simulink model "V2x_blockset"  (Simulink 7.6)
settings: Solver=ode45  StartTime=0.0  StopTime=10.0  RelTol=1e-3
undefined symbols (not defined in the file or in its folder): intmax, Newton, Raphson
libraries: simulink x53
(part 3 of 3)

== system V2x_blockset/Traffic Controller/Traffic signs and  traffic lights controller/Enabled Subsystem/distance condition/If Action Subsystem1 ==
  headway time : Inport
  d2 : Inport  Port=2
  Action Port : ActionPort  PropagateVarSize=During execution
  Add : Sum
  Gain : Gain  Gain=0
  t2 : Outport
  wires:
  Add/1 -> t2/1
  headway time/1 -> Add/2
  Gain/1 -> Add/1
  d2/1 -> Gain/1

== system V2x_blockset/Traffic Controller/Traffic signs and  traffic lights controller/Enabled Subsystem/major object selection lights/If Action Subsystem ==
  cond : Inport
  messagesID : Inport  Port=2
  traffic lights priorities : Inport  Port=3
  Action Port : ActionPort  PropagateVarSize=During execution
  Reshape1 : Reshape  OutputDimensionality=Column vector (2-D)
  Reshape2 : Reshape  OutputDimensionality=Column vector (2-D)
  Reshape3 : Reshape  OutputDimensionality=Column vector (2-D)
  Selector : Selector  NumberOfDimensions=2  InputPortWidth=3  IndexOptions=Index vector (port),Index vector (dialog)  Indices=[1 3],1  OutputSizes=1,1
  Selector1 : Selector  NumberOfDimensions=2  InputPortWidth=3  IndexOptions=Index vector (port),Index vector (dialog)  Indices=[1 3],1  OutputSizes=1,1
  While Iterator Subsystem : Subsystem  TreatAsAtomicUnit=on
  Message : Outport  InitialOutput=0
  Priority : Outport  Port=2  InitialOutput=0
  wires:
  Selector1/1 -> Priority/1
  Reshape3/1 -> Selector1/1
  traffic lights priorities/1 -> Reshape3/1
  messagesID/1 -> Reshape2/1
  While Iterator Subsystem/1(idx) -> Selector1/2, Selector/2
  Reshape2/1 -> Selector/1
  Reshape1/1 -> While Iterator Subsystem/1(cond)
  Selector/1 -> Message/1
  cond/1 -> Reshape1/1

== system V2x_blockset/Traffic Controller/Traffic signs and  traffic lights controller/Enabled Subsystem/major object selection lights/If Action Subsystem1 ==
  Action Port : ActionPort  PropagateVarSize=During execution
  Constant1 : Constant  Value=0
  Constant2 : Constant  Value=0
  Message : Outport  InitialOutput=0
  Priority : Outport  Port=2  InitialOutput=0
  wires:
  Constant2/1 -> Priority/1
  Constant1/1 -> Message/1

== system V2x_blockset/Traffic Controller/Traffic signs and  traffic lights controller/Enabled Subsystem/major object selection lights/Traffic Lights Warning ==
  trafficLightPriority : Inport
  Data Type Conversion : DataTypeConversion
  Logical Operator : Logic  Operator=OR  AllPortsSameDT=off  OutDataTypeStr=boolean
  if Orange light : simulink/Logic and Bit Operations/Compare To Constant  SystemSampleTime=-1  relop===  const=2  LogicOutDataTypeMode=uint8  ZeroCross=off
  if Red light : simulink/Logic and Bit Operations/Compare To Constant  SystemSampleTime=-1  relop===  const=1  LogicOutDataTypeMode=uint8  ZeroCross=off
  Warning : Outport
  wires:
  trafficLightPriority/1 -> if Orange light/1, if Red light/1
  Data Type Conversion/1 -> Warning/1
  Logical Operator/1 -> Data Type Conversion/1
  if Red light/1 -> Logical Operator/2
  if Orange light/1 -> Logical Operator/1

== system V2x_blockset/Traffic Controller/Traffic signs and  traffic lights controller/Enabled Subsystem/major object selection signs/If Action Subsystem ==
  cond : Inport
  messagesID : Inport  Port=2
  hostVelocity : Inport  Port=3
  Action Port : ActionPort  PropagateVarSize=During execution
  Reshape1 : Reshape  OutputDimensionality=Column vector (2-D)
  Reshape2 : Reshape  OutputDimensionality=Column vector (2-D)
  Selector : Selector  NumberOfDimensions=2  InputPortWidth=3  IndexOptions=Index vector (port),Index vector (dialog)  Indices=[1 3],1  OutputSizes=1,1
  Selector1 : Selector  NumberOfDimensions=2  InputPortWidth=3  IndexOptions=Index vector (port),Index vector (dialog)  Indices=[1 3],1  OutputSizes=1,1
  Traffic signs warning : Subsystem
  While Iterator Subsystem : Subsystem  TreatAsAtomicUnit=on
  Warning : Outport
  Message : Outport  Port=2  InitialOutput=0
  wires:
  Selector1/1 -> Traffic signs warning/1(MessageID)
  Traffic signs warning/1(Warning) -> Warning/1
  hostVelocity/1 -> Traffic signs warning/2(hostVelocity)
  messagesID/1 -> Reshape2/1
  While Iterator Subsystem/1(idx) -> Selector1/2, Selector/2
  Reshape2/1 -> Selector1/1, Selector/1
  Reshape1/1 -> While Iterator Subsystem/1(cond)
  Selector/1 -> Message/1
  cond/1 -> Reshape1/1

== system V2x_blockset/Traffic Controller/Traffic signs and  traffic lights controller/Enabled Subsystem/major object selection signs/If Action Subsystem1 ==
  Action Port : ActionPort  PropagateVarSize=During execution
  Constant1 : Constant  Value=0
  Constant2 : Constant  Value=0
  Warning : Outport  InitialOutput=0
  Message : Outport  Port=2  InitialOutput=0
  wires:
  Constant2/1 -> Warning/1
  Constant1/1 -> Message/1

== system V2x_blockset/Traffic Controller/Traffic signs and  traffic lights controller/Enabled Subsystem/orientation condition/to local reference system ==
  rotZ : Inport
  dX : Inport  Port=2
  dY : Inport  Port=3
  Add : Sum
  Add1 : Sum  Inputs=+-
  Product{,1..3} (4 alike) : Product  RndMeth=Zero
  Trigonometric Function : Trigonometry
  Trigonometric Function1 : Trigonometry  Operator=cos
  dy : Outport
  dx : Outport  Port=2
  wires:
  Add1/1 -> dy/1
  Add/1 -> dx/1
  Product3/1 -> Add1/2
  Product2/1 -> Add1/1
  Product/1 -> Add/2
  Product1/1 -> Add/1
  dY/1 -> Product2/2, Product1/2
  Trigonometric Function/1 -> Product3/1, Product1/1
  dX/1 -> Product3/2, Product/2
  Trigonometric Function1/1 -> Product2/1, Product/1
  rotZ/1 -> Trigonometric Function1/1, Trigonometric Function/1

== system V2x_blockset/Traffic Controller/Traffic signs and  traffic lights controller/Enabled Subsystem/right road side condition/to local reference system ==
  rotZ : Inport
  dX : Inport  Port=2
  dY : Inport  Port=3
  Add1 : Sum  Inputs=+-
  Product2 : Product  RndMeth=Zero
  Product3 : Product  RndMeth=Zero
  Trigonometric Function : Trigonometry
  Trigonometric Function1 : Trigonometry  Operator=cos
  dy : Outport
  wires:
  rotZ/1 -> Trigonometric Function/1, Trigonometric Function1/1
  Trigonometric Function1/1 -> Product2/1
  dX/1 -> Product3/2
  Trigonometric Function/1 -> Product3/1
  dY/1 -> Product2/2
  Product2/1 -> Add1/1
  Product3/1 -> Add1/2
  Add1/1 -> dy/1

== system V2x_blockset/Traffic Controller/Intersection warning controller/Enabled Subsystem/Intersection/Closest crossing selection/GPS to XYZ difference (vectorized) ==
  hostLat : Inport
  hostLong : Inport  Port=2
  hostAlt : Inport  Port=3
  lat : Inport  Port=4
  long : Inport  Port=5
  alt : Inport  Port=6
  Add : Sum  Inputs=+-
  Add1 : Sum  Inputs=+-
  Add2 : Sum  Inputs=+-
  Add3 : Sum  Inputs=+++
  Product{,1..4} (5 alike) : Product  RndMeth=Zero
  d2r : Gain  Gain=pi/180
  d2r1 : Gain  Gain=pi/180
  mean Earth radius (latitudal) : Constant  Value=6335439.8775
  mean Earth radius (longitudal) : Constant  Value=6378137.55
  dist_sq : Outport
  wires:
  lat/1 -> Add/1
  hostLat/1 -> Add/2
  long/1 -> Add1/1
  hostLong/1 -> Add1/2
  alt/1 -> Add2/1
  hostAlt/1 -> Add2/2
  Add/1 -> d2r/1
  Add1/1 -> d2r1/1
  d2r/1 -> Product2/1
  d2r1/1 -> Product1/1
  mean Earth radius (longitudal)/1 -> Product1/2
  mean Earth radius (latitudal)/1 -> Product2/2
  Product2/1 -> Product/1, Product/2
  Product1/1 -> Product3/1, Product3/2
  Add2/1 -> Product4/2, Product4/1
  Product/1 -> Add3/1
  Product3/1 -> Add3/2
  Product4/1 -> Add3/3
  Add3/1 -> dist_sq/1

== system V2x_blockset/Traffic Controller/Intersection warning controller/Enabled Subsystem/Intersection/Closest crossing selection/If Action Subsystem ==
  min : Inport
  dist_sq : Inport  Port=2
  GPS lat1 : Inport  Port=3
  GPS long1 : Inport  Port=4
  GPS alt1 : Inport  Port=5
  Action Port : ActionPort  PropagateVarSize=During execution
  Product7 : Product  RndMeth=Zero
  Product8 : Product  RndMeth=Zero
  Product9 : Product  RndMeth=Zero
  Relational Operator3 : RelationalOperator  Operator===  OutDataTypeStr=boolean
  Sum6 : Sum  Inputs=+
  Sum7 : Sum  Inputs=+
  Sum8 : Sum  Inputs=+
  GPS lat : Outport  InitialOutput=0
  GPS long : Outport  Port=2  InitialOutput=0
  GPS alt : Outport  Port=3  InitialOutput=0
  wires:
  min/1 -> Relational Operator3/1
  dist_sq/1 -> Relational Operator3/2
  Relational Operator3/1 -> Product7/1, Product8/1, Product9/1
  GPS lat1/1 -> Product7/2
  GPS long1/1 -> Product8/2
  GPS alt1/1 -> Product9/2
  Product7/1 -> Sum6/1
  Product8/1 -> Sum7/1
  Product9/1 -> Sum8/1
  Sum6/1 -> GPS lat/1
  Sum7/1 -> GPS long/1
  Sum8/1 -> GPS alt/1

== system V2x_blockset/Traffic Controller/Intersection warning controller/Enabled Subsystem/Intersection/Closest crossing selection/If Action Subsystem1 ==
  Action Port : ActionPort  PropagateVarSize=During execution
  Constant : Constant  Value=0
  Constant1 : Constant  Value=0
  Constant2 : Constant  Value=0
  GPS lat : Outport  InitialOutput=0
  GPS long : Outport  Port=2  InitialOutput=0
  GPS alt : Outport  Port=3  InitialOutput=0
  wires:
  Constant/1 -> GPS lat/1
  Constant1/1 -> GPS long/1
  Constant2/1 -> GPS alt/1

== system V2x_blockset/Traffic Controller/Intersection warning controller/Enabled Subsystem/Intersection/Intersection collision warning controller/For Each Subsystem ==
  actorType : Inport  PortDimensions=1  Partition=on  PartitionDimension=1  PartitionWidth=1
  WM : Inport  Port=2  Partition=off
  Rcross : Inport  Port=3  Partition=off
  target range : Inport  Port=4  Partition=on  PartitionDimension=1  PartitionWidth=1
  target angle : Inport  Port=5  Partition=on  PartitionDimension=1  PartitionWidth=1
  target intention : Inport  Port=6  Partition=on  PartitionDimension=1  PartitionWidth=1
  target heading : Inport  Port=7  Partition=on  PartitionDimension=1  PartitionWidth=1
  targetVelocity : Inport  Port=8  PortDimensions=1  Partition=on  PartitionDimension=1  PartitionWidth=1
  For Each : ForEach  DisableCoverage=on  IndexMode=One-based
  If : If  NumInputs=2  IfExpression=(u1==1 | u1==2 | u1 ==3) & (u2~=0)
  If Action Subsystem : Subsystem  TreatAsAtomicUnit=on
  If Action Subsystem1 : Subsystem  TreatAsAtomicUnit=on
  Merge : Merge
  Merge1 : Merge
  Merge2 : Merge
  warning left lane : Outport  ConcatenationDimension=1
  warning straight lane : Outport  Port=2  ConcatenationDimension=1
  warning right lane : Outport  Port=3  ConcatenationDimension=1
  wires:
  actorType/1 -> If/1
  If/1 -> If Action Subsystem/Action
  If/2 -> If Action Subsystem1/Action
  WM/1 -> If Action Subsystem/1(WM)
  Rcross/1 -> If Action Subsystem/2(Rcross)
  target range/1 -> If Action Subsystem/3(target range)
  target angle/1 -> If Action Subsystem/4(target angle)
  target intention/1 -> If Action Subsystem/5(target intention)
  target heading/1 -> If Action Subsystem/6(target heading)
  If Action Subsystem/1(warning left lane) -> Merge/1
  If Action Subsystem/2(warning straight lane) -> Merge1/1
  If Action Subsystem/3(warning right lane) -> Merge2/1
  If Action Subsystem1/1(warning left lane) -> Merge/2
  If Action Subsystem1/2(warning straight lane) -> Merge1/2
  If Action Subsystem1/3(warning right lane) -> Merge2/2
  Merge/1 -> warning left lane/1
  Merge1/1 -> warning straight lane/1
  Merge2/1 -> warning right lane/1
  targetVelocity/1 -> If/2

== system V2x_blockset/Traffic Controller/Intersection warning controller/Enabled Subsystem/Intersection/Intersection collision warning controller/host intention translation ==
  host intention : Inport
  Bias : Bias  Bias=2
  Multiport Switch : MultiPortSwitch  zeroidx=off
  left_turning : Constant  Value=[0 1 1 1 1 1 0 1 1]
  right_turning : Constant  Value=[0 1 0 0 0 1 0 0 0]
  straight : Constant  Value=[0 1 1 0 0 1 1 1 1]
  WM : Outport
  wires:
  right_turning/1 -> Multiport Switch/4
  straight/1 -> Multiport Switch/3
  left_turning/1 -> Multiport Switch/2
  host intention/1 -> Bias/1
  Bias/1 -> Multiport Switch/1
  Multiport Switch/1 -> WM/1

== system V2x_blockset/Traffic Controller/Traffic signs and  traffic lights controller/Enabled Subsystem/major object selection lights/If Action Subsystem/While Iterator Subsystem ==
  cond : Inport
  Compare To Zero : simulink/Logic and Bit Operations/Compare To Zero  SystemSampleTime=-1  relop===  LogicOutDataTypeMode=uint8  ZeroCross=off
  Selector : Selector  NumberOfDimensions=2  InputPortWidth=3  IndexOptions=Index vector (port),Index vector (dialog)  Indices=[1 3],1  OutputSizes=1,1
  While Iterator : WhileIterator  MaxIters=-1  WhileBlockType=do-while  ShowIterationPort=on  OutputDataType=double
  idx : Outport
  wires:
  Selector/1 -> Compare To Zero/1
  cond/1 -> Selector/1
  While Iterator/1 -> idx/1, Selector/2
  Compare To Zero/1 -> While Iterator/1

== system V2x_blockset/Traffic Controller/Traffic signs and  traffic lights controller/Enabled Subsystem/major object selection signs/If Action Subsystem/Traffic signs warning ==
  MessageID : Inport
  hostVelocity : Inport  Port=2
  Compare To Zero : simulink/Logic and Bit Operations/Compare To Zero  SystemSampleTime=-1  relop=>  LogicOutDataTypeMode=uint8  ZeroCross=off
  Data Type Conversion : DataTypeConversion
  Gain : Gain  Gain=3.6
  Logical Operator : Logic  AllPortsSameDT=off  OutDataTypeStr=boolean
  Relational Operator : RelationalOperator  Operator=<  OutDataTypeStr=boolean
  message to speed limit conversion : Bias  Bias=-1000
  Warning : Outport
  wires:
  Logical Operator/1 -> Data Type Conversion/1
  Compare To Zero/1 -> Logical Operator/1
  Relational Operator/1 -> Logical Operator/2
  Gain/1 -> Relational Operator/2
  hostVelocity/1 -> Gain/1
  message to speed limit conversion/1 -> Compare To Zero/1, Relational Operator/1
  MessageID/1 -> message to speed limit conversion/1
  Data Type Conversion/1 -> Warning/1

== system V2x_blockset/Traffic Controller/Traffic signs and  traffic lights controller/Enabled Subsystem/major object selection signs/If Action Subsystem/While Iterator Subsystem ==
  cond : Inport
  Compare To Zero : simulink/Logic and Bit Operations/Compare To Zero  SystemSampleTime=-1  relop===  LogicOutDataTypeMode=uint8  ZeroCross=off
  Selector : Selector  NumberOfDimensions=2  InputPortWidth=3  IndexOptions=Index vector (port),Index vector (dialog)  Indices=[1 3],1  OutputSizes=1,1
  While Iterator : WhileIterator  MaxIters=-1  WhileBlockType=do-while  ShowIterationPort=on  OutputDataType=double
  idx : Outport
  wires:
  Selector/1 -> Compare To Zero/1
  cond/1 -> Selector/1
  While Iterator/1 -> idx/1, Selector/2
  Compare To Zero/1 -> While Iterator/1

== system V2x_blockset/Traffic Controller/Intersection warning controller/Enabled Subsystem/Intersection/Intersection collision warning controller/For Each Subsystem/If Action Subsystem ==
  WM : Inport
  Rcross : Inport  Port=2
  target range : Inport  Port=3
  target angle : Inport  Port=4
  target intention : Inport  Port=5
  target heading : Inport  Port=6
  Action Port : ActionPort
  Decision Algorithm : Stateflow chart  TreatAsAtomicUnit=on
  warning left lane : Outport  InitialOutput=false(1)
  warning straight lane : Outport  Port=2  InitialOutput=false(1)
  warning right lane : Outport  Port=3  InitialOutput=false(1)
  wires:
  Decision Algorithm/1(wLeft) -> warning left lane/1
  Rcross/1 -> Decision Algorithm/2(Rcross)
  target range/1 -> Decision Algorithm/3(range)
  Decision Algorithm/2(wStraight) -> warning straight lane/1
  target angle/1 -> Decision Algorithm/4(angle)
  target intention/1 -> Decision Algorithm/5(intention)
  Decision Algorithm/3(wRight) -> warning right lane/1
  target heading/1 -> Decision Algorithm/6(heading)
  WM/1 -> Decision Algorithm/1(WM)

== system V2x_blockset/Traffic Controller/Intersection warning controller/Enabled Subsystem/Intersection/Intersection collision warning controller/For Each Subsystem/If Action Subsystem1 ==
  Action Port : ActionPort
  Constant : Constant  Value=false(1)
  Constant1 : Constant  Value=false(1)
  Constant2 : Constant  Value=false(1)
  warning left lane : Outport  InitialOutput=false(1)
  warning straight lane : Outport  Port=2  InitialOutput=false(1)
  warning right lane : Outport  Port=3  InitialOutput=false(1)
  wires:
  Constant/1 -> warning left lane/1
  Constant1/1 -> warning straight lane/1
  Constant2/1 -> warning right lane/1

== matlab function light generator/Lights generator ==
  data: red_time input double; lightID output double; yellow_time input double; green_time input double; time input double; time_delay input double; last_time input double; red output double; yellow output double; green output double; light_time output double; last_time_out output double
function [lightID, red, yellow, green, light_time, last_time_out] = fcn(red_time, yellow_time, green_time, time, time_delay, last_time)
%#eml
time2 = time - last_time + time_delay;
if ((time2) <= green_time)
    green = 1;
    yellow = 0;
    red = 0;
    lightID = 3;
    last_time_out = last_time;
    light_time = green_time - time2;
elseif((time2) <= (green_time+yellow_time))
    green = 0;
    yellow = 1;
    red = 0;
    lightID = 2;
    last_time_out = last_time;
    light_time = yellow_time - (time2 - green_time);
elseif((time2) <= (green_time+yellow_time + red_time - yellow_time))
    green = 0;
    yellow = 0;
    red = 1;
    lightID = 1;
    last_time_out = last_time;
    light_time = red_time - (time2 - green_time - yellow_time);
elseif((time2) <= (green_time+yellow_time + red_time))
    green = 0;
    yellow = 1;
    red = 1;
    lightID = 1;
    last_time_out = last_time;
    light_time = red_time - (time2 - green_time - yellow_time);
else
    green = 1;
    yellow = 0;
    red = 0;
    lightID = 3;
    last_time_out = time + time_delay;
    light_time = green_time - (time2 - green_time - yellow_time - red_time);
end

== stateflow chart Traffic Controller/Intersection warning controller/Enabled Subsystem/Intersection/Intersection collision warning controller/For Each Subsystem/If Action Subsystem/Decision Algorithm ==
  state controller
    state Lane3
      state Straight
        en: wRight=WM[8];
      state RightTurn
        en: wRight=WM[7];
      state LeftTurn
        en: wRight=WM[9];
      (junction 36) -> controller.Lane3.LeftTurn [order 2] : [intention<0]
      (junction 36) -> controller.Lane3.Straight [order 3] : [intention==0]
      (default) -> (junction 36) [order 1]
      (default) -> controller.Lane3.Straight [order 2]
      (junction 36) -> controller.Lane3.RightTurn [order 1] : [intention>0]
    state Lane2
      state RightTurn
        en: wStraight=WM[4];
      state LeftTurn
        en: wStraight=WM[6];
      state Straight
        en: wStraight=WM[5];
      (junction 35) -> controller.Lane2.Straight [order 2] : [intention==0]
      (default) -> controller.Lane2.Straight [order 2]
      (junction 35) -> controller.Lane2.RightTurn [order 3] : [intention>0]
      (junction 35) -> controller.Lane2.LeftTurn [order 1] : [intention<0]
      (default) -> (junction 35) [order 1]
    state Lane1
      state Straight
        en: wLeft=WM[2];
      state LeftTurn
        en: wLeft=WM[3];
      state RightTurn
        en: wLeft=WM[1];
      (junction 34) -> controller.Lane1.RightTurn [order 3] : [intention>0]
      (junction 34) -> controller.Lane1.LeftTurn [order 1] : [intention<0]
      (junction 34) -> controller.Lane1.Straight [order 2] : [intention==0]
      (default) -> controller.Lane1.Straight [order 2]
      (default) -> (junction 34) [order 1]
    state Enter
    controller.Lane1.LeftTurn -> Enter
    controller.Lane3.RightTurn -> Enter
    (default) -> Enter : {wLeft=0;
        | wStraight=0;
        | wRight=0;}
    controller.Lane3.Straight -> Enter
    controller.Lane3.LeftTurn -> Enter
    Enter -> Enter [order 4] : {wLeft=0;
        | wStraight=0;
        | wRight=0;}
    controller.Lane1.RightTurn -> Enter
    Enter -> Lane3 [order 2] : [angle>-90 && angle<-45 && range<Rcross...
        | && (heading>45 && heading<135)]
    controller.Lane1.Straight -> Enter
    controller.Lane2.RightTurn -> Enter
    controller.Lane2.LeftTurn -> Enter
    Enter -> Lane2 [order 1] : [angle>0 && angle<45 && range<Rcross...
        | && heading>135 && heading<225]
    Enter -> Lane1 [order 3] : [angle>90 && angle<135 && range<Rcross...
        | && heading>225 && heading<315]
    controller.Lane2.Straight -> Enter
  data: WM input double size=9; Rcross input double; range input double; angle input double; intention input double; heading input double; wLeft output boolean size=1 =false(1); wStraight output boolean size=1 =false(1); wRight output boolean size=1 =false(1)

== matlab function Traffic Controller/Intersection warning controller/Enabled Subsystem/sort using ID/Embedded MATLAB Function ==
  data: y output double; ids input double
function y = fcn(ids)
% Sorts ID vector

[~,y] = sort(ids,'descend');

end

== matlab function EEB/Angle mod ==
  data: u input double; y output double
function y = fcn(u)
%#eml

y = mod(u, 360);

== matlab function Rx_Noise/For Iterator Subsystem/Embedded MATLAB Function ==
  data: CAM input double; CAM_o output double size=[5, 16]; i input double; NoMM input double; tmp_in input double; tmp_out output double
function [CAM_o, tmp_out] = con(CAM, i, NoMM, tmp_in)
%#eml
CAM_o = CAM;
tmp_out = tmp_in;
if (CAM(i, 3) ~= 0)
    if (mod(tmp_in(i), NoMM+1) ~= 0)
        CAM_o(i, :) = zeros(1, 16);
    end
    tmp_out(i) = tmp_in(i)+1;
end

== stateflow chart EEB/EEBL ==
  state EEBL [parallel]
    settings: executionOrder=1
    state vForward
      (junction 119) -> (junction 115) : {bend = 1;}
      (junction 111) -> (junction 116) [order 2] : {bend = 0;}
      (junction 113) -> (junction 133) [order 1] : [(abs(CAM_Heading[i]-selfHeading)<45 || abs(CAM_Heading[i]-selfHeading)>315) || bend == 1 ]
      (default) -> (junction 111)
      (junction 110) -> (junction 116)
      (junction 115) -> (junction 110)
      (junction 129) -> (junction 125) : {vForward = 0;}
      (junction 127) -> (junction 126) : {vForward = 1;}
      (junction 128) -> (junction 127) [order 1] : [((abs(vAngle-selfHeading)<45 || abs(vAngle-selfHeading)>315) && (abs(vDistance*sin(vAngle*d2r))<5.25)) || bend == 1]
      (junction 128) -> (junction 129) [order 2]
      (junction 130) -> (junction 128)
      (junction 132) -> (junction 129)
      (junction 131) -> (junction 130) [order 1] : [vDistance < 100 && (abs(selfGPSAltitude - CAM_GPSAltitude[i]) < 10)]
      (junction 131) -> (junction 132) [order 2]
      (junction 133) -> (junction 131)
      (junction 113) -> (junction 132) [order 2]
      (junction 118) -> (junction 119) [order 1] : [((abs(L/selfVelocity*selfYawRate + selfHeading - CAM_Heading[i]) < 45) || (abs(L/selfVelocity*selfYawRate + selfHeading - CAM_Heading[i]) > 315)) ]
      (junction 116) -> (junction 113)
      (junction 118) -> (junction 110) [order 2] : {bend = 2;}
      (junction 111) -> (junction 112) [order 1] : [((CAM_YawRate[i] > 2 || CAM_YawRate[i] <-2)  && (selfYawRate > 2 || selfYawRate < -2))]
      (junction 112) -> (junction 118) : {R1 = CAM_Velocity[i]/(CAM_YawRate[i]*d2r);
          | R2 = selfVelocity/(selfYawRate*d2r);
          | alfa = CAM_Heading[i]-selfHeading;
          | L = 2*d2r*180*R2*(alfa/360);}
    state dvBreaking
      (junction 122) -> (junction 120)
      (junction 123) -> (junction 121) : {vBreaking = 1;}
      (junction 121) -> (junction 122)
      (junction 124) -> (junction 122) [order 2]
      (junction 124) -> (junction 123) [order 1] : [ (vForward == 1 && CAM_Acceleration[i] < -brakingWarning)]
      (default) -> (junction 124) : /* Velocity */
    state VehicleAngleandDistance
      state vDistance [parallel]
        settings: executionOrder=2
        (junction 140) -> (junction 139) : {c=2*atan2(sqrt(a), sqrt(1-a));}
        (junction 139) -> (junction 114) : {vDistance = 6371000*c;}
        (default) -> (junction 140) : {a = (sin((CAM_GPSLatitude[i]*d2r-selfGPSLatitude*d2r)/2 ))^2+ cos(selfGPSLatitude*d2r)*cos(CAM_GPSLatitude[i]*d2r)*(sin((CAM_GPSLongitude[i]*d2r-selfGPSLongitude*d2r)/2))^2;}
      state vAngle [parallel]
        settings: executionOrder=1
        (default) -> (junction 117) : {vAngle = (atan2(CAM_GPSLatitude[i]-selfGPSLatitude, CAM_GPSLongitude[i] - selfGPSLongitude))/d2r;}
    state Breaking
      (default) -> (junction 135)
      (junction 135) -> (junction 134) : {Breaking = vBreaking;}
    vForward -> dvBreaking
    VehicleAngleandDistance -> vForward
    (junction 136) -> (junction 138) : {i++;}
    Breaking -> (junction 137)
    (junction 137) -> (junction 138) : {i = 0;
        | vBreaking = 0;
        | vForward = 0;}
    dvBreaking -> (junction 136)
    (junction 138) -> Breaking [order 2]
    (junction 138) -> VehicleAngleandDistance [order 1] : [i < CAM_Size && vBreaking != 1 ]
    (default) -> (junction 138) : {i =0;
        | vForward = 0;}
  note: EEB works with continous signal and checks deceleration of vehicles ahead
  data: a local double; alfa local double; bend local double; c local double; i local double; L local double; vAngle local double; vDistance local double; vForward local double; R1 local double; R2 local double; selfGPSLatitude input double; selfGPSLongitude input double; selfGPSAltitude input double; selfHeading input double; selfVelocity input double; selfYawRate input double; CAM_Velocity input double; CAM_Acceleration input double; CAM_YawRate input double; CAM_GPSLatitude input double; CAM_GPSLongitude input double; CAM_GPSAltitude input double; CAM_Heading input double; CAM_Size input double; d2r constant double =pi()/180; Breaking output double; vBreaking local double; brakingWarning constant double =0.4*9.81

== matlab function Rx_Noise/Embedded MATLAB Function ==
  data: CAM_warning input double; CAM output double; CAM_messageID input double; CAM_vehicleID input double; CAM_vehicleType input double; CAM_publicVehicleType input double; CAM_lightBarInUse input double; CAM_sireneInUse input double; CAM_velocity input double; CAM_acceleration input double; CAM_yawRate input double; CAM_turnAdvice input double; CAM_trafficLightPriority input double; CAM_GPSlat input double; CAM_GPSlong input double; CAM_GPSalt input double; CAM_rotZ input double
function CAM = fcn(CAM_warning, CAM_messageID, CAM_vehicleID, CAM_vehicleType, CAM_publicVehicleType, CAM_lightBarInUse, CAM_sireneInUse, CAM_velocity, CAM_acceleration, CAM_yawRate, CAM_turnAdvice, CAM_trafficLightPriority, CAM_GPSlat, CAM_GPSlong, CAM_GPSalt, CAM_rotZ)
%#eml

CAM = [CAM_warning, CAM_messageID, CAM_vehicleID, CAM_vehicleType, CAM_publicVehicleType, CAM_lightBarInUse, CAM_sireneInUse, CAM_velocity, CAM_acceleration, CAM_yawRate, CAM_turnAdvice, CAM_trafficLightPriority, CAM_GPSlat, CAM_GPSlong, CAM_GPSalt, CAM_rotZ];

== matlab function Rx_Noise/Embedded MATLAB Function1 ==
  data: CAM_warning output double; CAM input double; CAM_messageID output double; CAM_vehicleID output double; CAM_vehicleType output double; CAM_publicVehicleType output double; CAM_lightBarInUse output double; CAM_sireneInUse output double; CAM_velocity output double; CAM_acceleration output double; CAM_yawRate output double; CAM_turnAdvice output double; CAM_trafficLightPriority output double; CAM_GPSlat output double; CAM_GPSlong output double; CAM_GPSalt output double; CAM_rotZ output double
function [CAM_warning, CAM_messageID, CAM_vehicleID, CAM_vehicleType, CAM_publicVehicleType, CAM_lightBarInUse, CAM_sireneInUse, CAM_velocity, CAM_acceleration, CAM_yawRate, CAM_turnAdvice, CAM_trafficLightPriority, CAM_GPSlat, CAM_GPSlong, CAM_GPSalt, CAM_rotZ] = fcn(CAM)
%#eml

CAM_warning = CAM(:, 1);
CAM_messageID = CAM(:, 2); 
CAM_vehicleID = CAM(:, 3);
CAM_vehicleType = CAM(:, 4);
CAM_publicVehicleType = CAM(:, 5);
CAM_lightBarInUse = CAM(:, 6);
CAM_sireneInUse = CAM(:, 7);
CAM_velocity = CAM(:, 8);
CAM_acceleration = CAM(:, 9);
CAM_yawRate = CAM(:, 10);
CAM_turnAdvice = CAM(:, 11);
CAM_trafficLightPriority = CAM(:, 12);
CAM_GPSlat = CAM(:, 13);
CAM_GPSlong = CAM(:, 14);
CAM_GPSalt = CAM(:, 15);
CAM_rotZ = CAM(:, 16);

== matlab function GLOSA/Embedded MATLAB Function ==
  data: u input double; y output double
function y = fcn(u)
%#eml

y = mod(u, 360);

== stateflow chart GLOSA/GLOSA ==
  state GLOSA [parallel]
    settings: executionOrder=1
    state dvVelocity
      (default) -> (junction 337) : /* Velocity */
      (junction 337) -> (junction 339) [order 1] : [ (vForward == 1)]
      (junction 339) -> (junction 349) : {dvVelocity = CAM_Velocity[i];}
          | /* If car is at the front desired velocity if cars are set to its value */
      (junction 337) -> (junction 283) [order 2] : {dvVelocity = desiredVelocity;}
      (junction 349) -> (junction 283)
      (junction 283) -> (junction 350)
    state AngleandDistance
      state vDistance [parallel]
        settings: executionOrder=2
        (junction 331) -> (junction 330) : {Distance = 6371000*c;}
            | /*Calculate distance to the object */
        (default) -> (junction 332) : {a = (sin((CAM_GPSLatitude[i]*d2r-selfGPSLatitude*d2r)/2 ))^2+ cos(selfGPSLatitude*d2r)*cos(CAM_GPSLatitude[i]*d2r)*(sin((CAM_GPSLongitude[i]*d2r-selfGPSLongitude*d2r)/2))^2;}
        (junction 332) -> (junction 331) : {c=2*atan2(sqrt(a), sqrt(1-a));}
      state vAngle [parallel]
        settings: executionOrder=1
        (default) -> (junction 333) : {Angle = (atan2(CAM_GPSLatitude[i]-selfGPSLatitude, CAM_GPSLongitude[i] - selfGPSLongitude))/d2r;}
            | /* Calculate angle to the object */
    state diVelocity
      (default) -> (junction 304) : /* Velocity */
      (junction 285) -> (junction 338)
      (junction 304) -> (junction 303) [order 1] : [ (iForward == 1)]
      (junction 304) -> (junction 285) [order 2] : {diVelocity = desiredVelocity;}
      (junction 303) -> (junction 336) : {diVelocity = (CAM_message[i] - 1000) /3.6;}
          | /* If sign is foreward, set desired infrastructure velocity to its limit */
      (junction 336) -> (junction 285)
    state vForward
      (junction 289) -> (junction 295) [order 1] : [((CAM_YawRate[i] > 2 || CAM_YawRate[i] <-2)  && (selfYawRate > 2 || selfYawRate < -2))]
      (junction 295) -> (junction 319) : {R1 = CAM_Velocity[i]/(CAM_YawRate[i]*d2r);
          | R2 = selfVelocity/(selfYawRate*d2r);
          | alfa = CAM_Heading[i]-selfHeading;
          | L = 2*d2r*180*R2*(alfa/360);}
      (junction 356) -> (junction 341)
      (junction 340) -> (junction 356) : {bend = 1;}
          | /* Cars are on the same bent if both have non-zero yaw rate and estimated agle at detected distance of the host car is similar to the angle of detected vehicle */
      (junction 319) -> (junction 341) [order 2] : {bend = 2;}
      (junction 279) -> (junction 282)
      (junction 293) -> (junction 280) [order 2]
      (junction 341) -> (junction 294)
      (junction 294) -> (junction 293)
      (junction 282) -> (junction 280) [order 2]
      (default) -> (junction 289)
      (junction 286) -> (junction 287) [order 1] : [abs((Angle-selfHeading)%%360)<45 || abs((Angle-selfHeading)%%360)>315 || bend == 1]
      (junction 335) -> (junction 327) : {vForward = 0;}
      (junction 287) -> (junction 288) : {vForward = 1;}
          | /* Car is at the front if it will be reached in 2s and angles of cars are similar or they are on the bend */
      (junction 293) -> (junction 279) [order 1] : [(abs(CAM_Heading[i]-selfHeading)<45 || abs(CAM_Heading[i]-selfHeading)>315) || bend == 1 ]
      (junction 286) -> (junction 335) [order 2]
      (junction 282) -> (junction 284) [order 1] : [Distance < 100 && (selfVelocity - CAM_Velocity[i]) > 0 &&((Distance / (selfVelocity - CAM_Velocity[i])) < 2) && (abs(selfGPSAltitude - CAM_GPSAltitude[i]) < 10)]
      (junction 289) -> (junction 294) [order 2] : {bend = 0;}
      (junction 284) -> (junction 286)
      (junction 280) -> (junction 335)
      (junction 319) -> (junction 340) [order 1] : [((abs(L/selfVelocity*selfYawRate + selfHeading - CAM_Heading[i]) < 45) || (abs(L/selfVelocity*selfYawRate + selfHeading - CAM_Heading[i]) > 315)) ]
    state Velocity
      (junction 309) -> (junction 307) [order 2]
      (junction 309) -> (junction 308) [order 1] : [(dvVelocity<diVelocity) && (dvVelocity < desiredVelocity) && (vForward == 1)]
      (junction 311) -> (junction 309)
      (junction 310) -> (junction 311)
      (junction 325) -> (junction 310) : {Velocity = diVelocity;}
          | /* When Velocity from the sign is smaller then actual velocity of the car, Desired host velocity is set to the sign limit */
      (junction 326) -> (junction 311) [order 2] : {Velocity = desiredVelocity;}
      (junction 326) -> (junction 325) [order 1] : [(diVelocity<desiredVelocity)]
      (default) -> (junction 326) : /* Velocity */
      (junction 308) -> (junction 306) : {Velocity = dvVelocity;}
          | /* When detected car hes smaller velocity then host car and sign limits, desired velocity of host car is set to velocity of detected car */
      (junction 307) -> (junction 305) : {Velocity = min(dvVelocity, diVelocity, dlVelocity, desiredVelocity);}
      (junction 306) -> (junction 307)
    state lForward
      note: IF condition1 THEN action1
          | ELSE action2
          | ENDIF
      (junction 346) -> (junction 291) : {lForward = 0;}
      (junction 362) -> (junction 292) : {lForward = 1;}
          | /* Light recognized as foreward one, when it is less then 500m away and Angle to it less then 45 deg.*/
      (junction 344) -> (junction 362) [order 1] : [abs((Angle-selfHeading) %% 360)<45 || abs((Angle-selfHeading)%% 360)>315]
      (junction 344) -> (junction 346) [order 2]
      (junction 359) -> (junction 342) [order 2]
      (junction 343) -> (junction 342) [order 2]
      (junction 348) -> (junction 344)
      (junction 358) -> (junction 343)
      (junction 343) -> (junction 348) [order 1] : [Distance < 500 && (abs(selfGPSAltitude - CAM_GPSAltitude[i]) < 10)]
      (junction 342) -> (junction 346)
      (junction 359) -> (junction 358) [order 1] : [abs(CAM_Heading[i]-selfHeading)<45 || abs(CAM_Heading[i]-selfHeading)>315]
      (default) -> (junction 359)
    state iForward
      note: IF condition1 THEN action1
          | ELSE action2
          | ENDIF
      (junction 281) -> (junction 328) [order 1] : [Distance < 20 && (abs(selfGPSAltitude - CAM_GPSAltitude[i]) < 10)]
      (junction 290) -> (junction 316) [order 1] : [abs((Angle-selfHeading)%%360)<45 || abs((Angle-selfHeading)%%360)>315]
      (junction 281) -> (junction 315) [order 2]
      (junction 316) -> (junction 317) : {iForward = 1;}
          | /* Sign recognized as foreward one, when it is less then 20m away and Angle to it less then 45 deg.*/
      (junction 315) -> (junction 329)
      (junction 328) -> (junction 290)
      (junction 329) -> (junction 318) : {iForward = 0;}
      (junction 290) -> (junction 329) [order 2]
      (junction 334) -> (junction 324) [order 1] : [abs(CAM_Heading[i]-selfHeading)<45 || abs(CAM_Heading[i]-selfHeading)>315]
      (default) -> (junction 334)
      (junction 324) -> (junction 281)
      (junction 334) -> (junction 315) [order 2]
    state dlVelocity
      (junction 322) -> (junction 320) : {dlVelocity = max((Distance-7)/(CAM_warning[i]+20), 0);}
          | /*dlVelocity = Distance/CAM_warning[i];}*/
      (junction 353) -> (junction 323) [order 2]
      (junction 357) -> (junction 360)
      (junction 361) -> (junction 357)
      (junction 351) -> (junction 357) [order 2] : {dlVelocity=desiredVelocity;}
      (junction 347) -> (junction 345)
      (junction 355) -> (junction 353) [order 2]
      (junction 320) -> (junction 361)
      (junction 323) -> (junction 322) [order 2]
      (junction 323) -> (junction 321) [order 1] : [TTL<CAM_warning[i]]
      (junction 355) -> (junction 354) [order 1] : [CAM_trafficLightPriority[i] == 3]
      (junction 321) -> (junction 345) : {dlVelocity= desiredVelocity;}
      (junction 297) -> (junction 347)
      (junction 345) -> (junction 320)
      (junction 354) -> (junction 297) : {dlVelocity=desiredVelocity;}
      (junction 296) -> (junction 347) : {dlVelocity = max((Distance-2)/(CAM_warning[i]+0.5), 0);}
      (junction 353) -> (junction 296) [order 1] : [CAM_trafficLightPriority[i] == 1]
      (default) -> (junction 351) : /* Velocity */
      (junction 351) -> (junction 352) [order 1] : [ lForward == 1]
      (junction 352) -> (junction 355) : {TTL = Distance/selfVelocity;
          | Light = CAM_trafficLightPriority[i];
          | Time = CAM_warning[i];}
    lForward -> dlVelocity
    (junction 299) -> AngleandDistance
    (default) -> (junction 298) : {i =0;
        | vForward = 0;
        | iForward = 0;}
    (junction 298) -> (junction 299) [order 1] : [(vForward ==0 || iForward == 0) && i < CAM_Size]
        |  /*till sign and vehicle aren't detected*/
    (junction 300) -> iForward [order 2] : [iForward == 0 && (CAM_vehicleType[i] == 14 || CAM_vehicleType[i] == 15) && CAM_message[i] > 1000]
        | /* If no traffic sign are detected and Velocity of the sign isn't 0 */
    (junction 302) -> (junction 298) : {i = 0;
        | vForward = 0;
        | iForward = 0;
        | lForward = 0;}
    (junction 312) -> (junction 298) : {i++;}
    (junction 300) -> (junction 301) [order 3]
    (junction 298) -> Velocity [order 2]
    (junction 301) -> vForward [order 1] : [vForward == 0 && CAM_vehicleType[i] != 0]
        | /* If there was no nearer car at the front and Vehicle Type ID isn't 0 */
    (junction 301) -> (junction 312) [order 2]
    iForward -> diVelocity
    Velocity -> (junction 302)
    vForward -> dvVelocity
    dvVelocity -> (junction 314)
    diVelocity -> (junction 314)
    (junction 313) -> (junction 312)
    (junction 314) -> (junction 313)
    AngleandDistance -> (junction 300)
    (junction 300) -> lForward [order 1] : [lForward == 0 && CAM_trafficLightPriority[i] !=0]
    dlVelocity -> (junction 314)
  note: GLOSA Algorithms Based on CAM signal changed to continous
  data: R1 local double; R2 local double; a local double; alfa local double; bend local double; c local double; diVelocity local double =100; dvVelocity local double =100; i local double; iForward local double; L local double; vForward local double; dlVelocity local double =100; selfHeading input double; selfGPSLongitude input double; selfGPSLatitude input double; selfGPSAltitude input double; selfYawRate input double; selfVelocity input double; CAM_warning input double; CAM_message input double; CAM_vehicleType input double; Velocity output double; CAM_Velocity input double; CAM_YawRate input double; CAM_trafficLightPriority input double; CAM_GPSLatitude input double; CAM_GPSLongitude input double; CAM_GPSAltitude input double; CAM_Heading input double; CAM_Size input double; d2r constant double =pi()/180; desiredVelocity input double; TTL local double; lForward output double; Angle local double; Distance local double; Time output double; Light output double

== matlab function GLOSA/vehicle CAM generator/For Iterator Subsystem/Continuous signal ==
  data: CAM input double; CAM_o output double; CAM_old input double; i input double; NoMM input double; tmp_in input double; tmp_out output double
function [CAM_o, tmp_out] = con(CAM, CAM_old, i, NoMM, tmp_in)
%linearization and number of missed frames control
CAM_o = zeros(1, 16);
tmp_out = tmp_in(i);
if (CAM(i, 3) ~= 0)
    if (mod(tmp_in(i), NoMM+1) == 0)
        CAM_o = CAM (i, :);
    end
    tmp_out = tmp_in(i)+1;
else
    CAM_o = CAM_old(i, :);
end

== matlab function GLOSA/vehicle CAM generator/Seperate signals ==
  data: CAM_warning output double; CAM input double; CAM_messageID output double; CAM_vehicleID output double; CAM_vehicleType output double; CAM_publicVehicleType output double; CAM_lightBarInUse output double; CAM_sireneInUse output double; CAM_velocity output double; CAM_acceleration output double; CAM_yawRate output double; CAM_turnAdvice output double; CAM_trafficLightPriority output double; CAM_GPSlat output double; CAM_GPSlong output double; CAM_GPSalt output double; CAM_rotZ output double
function [CAM_warning, CAM_messageID, CAM_vehicleID, CAM_vehicleType, CAM_publicVehicleType, CAM_lightBarInUse, CAM_sireneInUse, CAM_velocity, CAM_acceleration, CAM_yawRate, CAM_turnAdvice, CAM_trafficLightPriority, CAM_GPSlat, CAM_GPSlong, CAM_GPSalt, CAM_rotZ] = fcn(CAM)
%Seperate signals

CAM_warning = CAM(:, 1);
CAM_messageID = CAM(:, 2); 
CAM_vehicleID = CAM(:, 3);
CAM_vehicleType = CAM(:, 4);
CAM_publicVehicleType = CAM(:, 5);
CAM_lightBarInUse = CAM(:, 6);
CAM_sireneInUse = CAM(:, 7);
CAM_velocity = CAM(:, 8);
CAM_acceleration = CAM(:, 9);
CAM_yawRate = CAM(:, 10);
CAM_turnAdvice = CAM(:, 11);
CAM_trafficLightPriority = CAM(:, 12);
CAM_GPSlat = CAM(:, 13);
CAM_GPSlong = CAM(:, 14);
CAM_GPSalt = CAM(:, 15);
CAM_rotZ = CAM(:, 16);

== matlab function GLOSA/vehicle CAM generator/Signal Matrix create ==
  data: CAM_warning input double; CAM output double; CAM_messageID input double; CAM_vehicleID input double; CAM_vehicleType input double; CAM_publicVehicleType input double; CAM_lightBarInUse input double; CAM_sireneInUse input double; CAM_velocity input double; CAM_acceleration input double; CAM_yawRate input double; CAM_turnAdvice input double; CAM_trafficLightPriority input double; CAM_GPSlat input double; CAM_GPSlong input double; CAM_GPSalt input double; CAM_rotZ input double
function CAM = fcn(CAM_warning, CAM_messageID, CAM_vehicleID, CAM_vehicleType, CAM_publicVehicleType, CAM_lightBarInUse, CAM_sireneInUse, CAM_velocity, CAM_acceleration, CAM_yawRate, CAM_turnAdvice, CAM_trafficLightPriority, CAM_GPSlat, CAM_GPSlong, CAM_GPSalt, CAM_rotZ)
%Signal Matrix creation

CAM = [CAM_warning, CAM_messageID, CAM_vehicleID, CAM_vehicleType, CAM_publicVehicleType, CAM_lightBarInUse, CAM_sireneInUse, CAM_velocity, CAM_acceleration, CAM_yawRate, CAM_turnAdvice, CAM_trafficLightPriority, CAM_GPSlat, CAM_GPSlong, CAM_GPSalt, CAM_rotZ];

== matlab function EEB/vehicle CAM generator/Signal Matrix create ==
  data: CAM_warning input double; CAM output double; CAM_messageID input double; CAM_vehicleID input double; CAM_vehicleType input double; CAM_publicVehicleType input double; CAM_lightBarInUse input double; CAM_sireneInUse input double; CAM_velocity input double; CAM_acceleration input double; CAM_yawRate input double; CAM_turnAdvice input double; CAM_trafficLightPriority input double; CAM_GPSlat input double; CAM_GPSlong input double; CAM_GPSalt input double; CAM_rotZ input double
function CAM = fcn(CAM_warning, CAM_messageID, CAM_vehicleID, CAM_vehicleType, CAM_publicVehicleType, CAM_lightBarInUse, CAM_sireneInUse, CAM_velocity, CAM_acceleration, CAM_yawRate, CAM_turnAdvice, CAM_trafficLightPriority, CAM_GPSlat, CAM_GPSlong, CAM_GPSalt, CAM_rotZ)
%Signal Matrix creation

CAM = [CAM_warning, CAM_messageID, CAM_vehicleID, CAM_vehicleType, CAM_publicVehicleType, CAM_lightBarInUse, CAM_sireneInUse, CAM_velocity, CAM_acceleration, CAM_yawRate, CAM_turnAdvice, CAM_trafficLightPriority, CAM_GPSlat, CAM_GPSlong, CAM_GPSalt, CAM_rotZ];

== matlab function EEB/vehicle CAM generator/Seperate signals ==
  data: CAM_warning output double; CAM input double; CAM_messageID output double; CAM_vehicleID output double; CAM_vehicleType output double; CAM_publicVehicleType output double; CAM_lightBarInUse output double; CAM_sireneInUse output double; CAM_velocity output double; CAM_acceleration output double; CAM_yawRate output double; CAM_turnAdvice output double; CAM_trafficLightPriority output double; CAM_GPSlat output double; CAM_GPSlong output double; CAM_GPSalt output double; CAM_rotZ output double
function [CAM_warning, CAM_messageID, CAM_vehicleID, CAM_vehicleType, CAM_publicVehicleType, CAM_lightBarInUse, CAM_sireneInUse, CAM_velocity, CAM_acceleration, CAM_yawRate, CAM_turnAdvice, CAM_trafficLightPriority, CAM_GPSlat, CAM_GPSlong, CAM_GPSalt, CAM_rotZ] = fcn(CAM)
%Seperate signals

CAM_warning = CAM(:, 1);
CAM_messageID = CAM(:, 2); 
CAM_vehicleID = CAM(:, 3);
CAM_vehicleType = CAM(:, 4);
CAM_publicVehicleType = CAM(:, 5);
CAM_lightBarInUse = CAM(:, 6);
CAM_sireneInUse = CAM(:, 7);
CAM_velocity = CAM(:, 8);
CAM_acceleration = CAM(:, 9);
CAM_yawRate = CAM(:, 10);
CAM_turnAdvice = CAM(:, 11);
CAM_trafficLightPriority = CAM(:, 12);
CAM_GPSlat = CAM(:, 13);
CAM_GPSlong = CAM(:, 14);
CAM_GPSalt = CAM(:, 15);
CAM_rotZ = CAM(:, 16);

== matlab function EEB/vehicle CAM generator/For Iterator Subsystem/Continuous signal ==
  data: CAM input double; CAM_o output double; CAM_old input double; i input double; NoMM input double; tmp_in input double; tmp_out output double
function [CAM_o, tmp_out] = con(CAM, CAM_old, i, NoMM, tmp_in)
%linearization and number of missed frames control
CAM_o = zeros(1, 16);
tmp_out = tmp_in(i);
if (CAM(i, 3) ~= 0)
    if (mod(tmp_in(i), NoMM+1) == 0)
        CAM_o = CAM (i, :);
    end
    tmp_out = tmp_in(i)+1;
else
    CAM_o = CAM_old(i, :);
end
